simulink model "rockets_v2"  (R2020a)
settings: Solver=VariableStepAuto  StartTime=0.0  StopTime=10  RelTol=1e-3
undefined symbols (not defined in the file): Earth, F_z, length_rocket, mass_rocket, WGS84
libraries: shared6dof x1, aerolibtransform2 x1, aerolibfltsims x1, vrlib x1, sharedtransform x1
settings Model: PacingRate=0.890000  Creator=Benjamin_de_worsop  LastModifiedBy=Benjamin_de_worsop

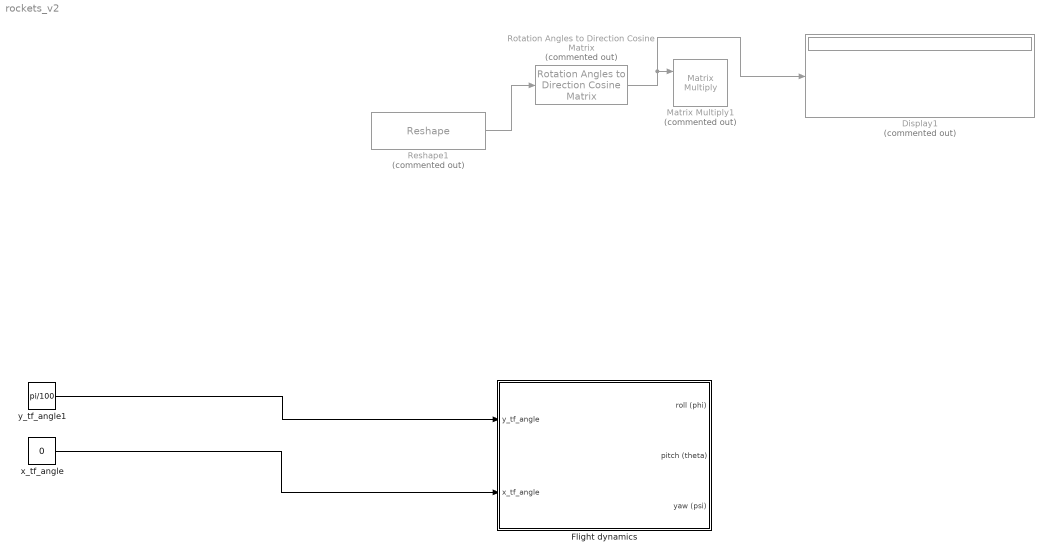
== system rockets_v2 ==
  Display1 : Display  Commented=on
  Flight dynamics : Subsystem
  Matrix Multiply1 : Product  Commented=on  Multiplication=Matrix(*)
  Reshape1 : Reshape  Commented=on  OutputDimensionality=Customize  OutputDimensions=[1, 3]
  Rotation Angles to Direction Cosine Matrix : sharedtransform/Rotation Angles to Direction Cosine Matrix  Commented=on  rotationOrder=YXZ  aMode=aMode
      settings: SourceProductBaseCode=AE,PW,MT,VE,VP
  x_tf_angle : Constant  Value=0
  y_tf_angle1 : Constant  Value=pi/100
  wires:
  Rotation Angles to Direction Cosine Matrix/1 -> Display1/1, Matrix Multiply1/1
  Reshape1/1 -> Rotation Angles to Direction Cosine Matrix/1
  y_tf_angle1/1 -> Flight dynamics/1(y_tf_angle)
  x_tf_angle/1 -> Flight dynamics/2(x_tf_angle)

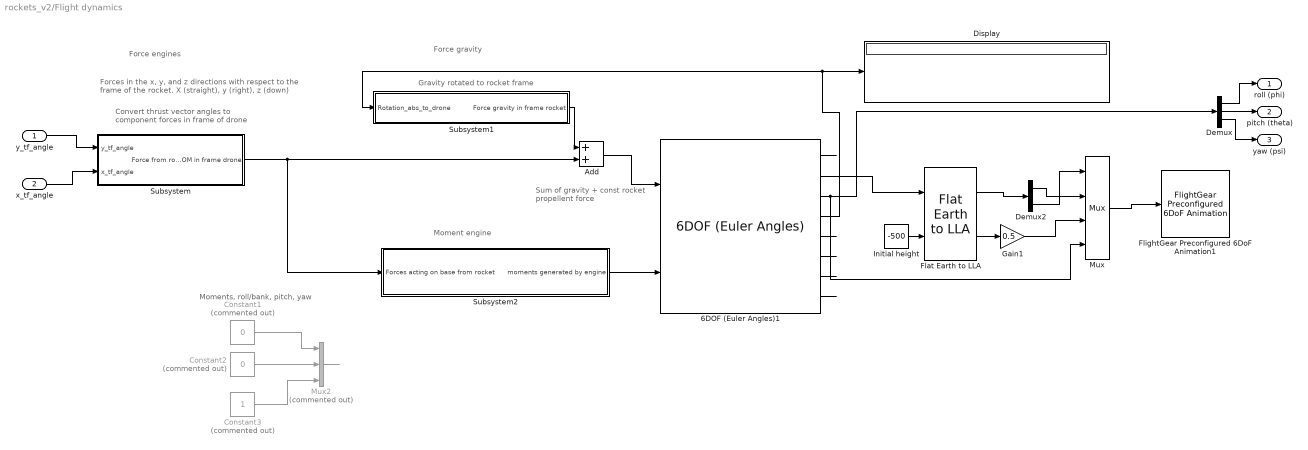
== system rockets_v2/Flight dynamics ==
  note: Convert thrust vector angles to component forces in frame of drone
  note: Moment engine
  note: Sum of gravity + const rocket propellent force
  note: Gravity rotated to rocket frame
  note: Forces in the x, y, and z directions with respect to the frame of the rocket. X (straight), y (right), z (down)
  note: Moments, roll/bank, pitch, yaw
  note: Force engines
  note: Force gravity
  y_tf_angle : Inport
  x_tf_angle : Inport  Port=2
  6DOF (Euler Angles)1 : shared6dof/6DOF (Euler Angles)  units=Metric (MKS)  mtype=Fixed  rep=Euler Angles  xme_0=[-122.482, 37.6655, 400]  Vm_0=[0 0 0]  eul_0=[0 0 0]  pm_0=[0 0 0]  mass_0=1  mass_e=0.5  mass_f=2.0  inertia=eye(3)  inertia_e=eye(3)  inertia_f=2*eye(3)  k_quat=1.0  vre_flag=on  abi_flag=off  aMode=0  xme_statename=''  Vm_statename=''  eul_statename=''  quat_statename=''  pm_statename=''  mass_statename=''
      settings: SourceProductBaseCode=AE,PW,MT,VE,VP
  Add : Sum
  Constant1 : Constant  Commented=on  Value=0
  Constant2 : Constant  Commented=on  Value=0
  Constant3 : Constant  Commented=on
  Demux : Demux  Outputs=3
  Demux2 : Demux  Outputs=2
  Display : Display
  Flat Earth to LLA : aerolibtransform2/Flat Earth to LLA  units=Metric (MKS)  ptype=Earth (WGS84)  F=1/298.257223563  R=6378137  refPosPort=off  LL0=[0 10]  psi=0
  FlightGear Preconfigured 6DoF Animation1 : aerolibfltsims/FlightGear Preconfigured 6DoF Animation  xFlightGearVersion=v2019.1  DestinationIpAddress=127.0.0.1  DestinationPort=5502  SampleTime=1/30  packetVersion=24
  Gain1 : Gain  Gain=0.5
  Initial height : Constant  Value=-500
  Mux : Mux
  Mux2 : Mux  Commented=on  Inputs=3
  Subsystem : Subsystem
  Subsystem1 : Subsystem
  Subsystem2 : Subsystem
  roll (phi) : Outport
  pitch (theta) : Outport  Port=2
  yaw (psi) : Outport  Port=3
  wires:
  Demux2/1 -> Mux/2
  Flat Earth to LLA/1 -> Demux2/1
  Gain1/1 -> Mux/3
  Demux2/2 -> Mux/1
  Subsystem/1(Force from rocket COM in frame drone) -> Add/2, Subsystem2/1(Forces acting on base from rocket)
  Initial height/1 -> Flat Earth to LLA/2
  6DOF (Euler Angles)1/8 -> ?
  6DOF (Euler Angles)1/6 -> ?
  Mux/1 -> FlightGear Preconfigured 6DoF Animation1/1
  Flat Earth to LLA/2 -> Gain1/1
  6DOF (Euler Angles)1/2 -> Flat Earth to LLA/1
  6DOF (Euler Angles)1/5 -> ?
  6DOF (Euler Angles)1/4 -> Display/1, Subsystem1/1(Rotation_abs_to_drone)
  6DOF (Euler Angles)1/3 -> Demux/1, Mux/4
  Subsystem2/1(moments generated by engine) -> 6DOF (Euler Angles)1/2
  x_tf_angle/1 -> Subsystem/2(x_tf_angle)
  Constant1/1 -> Mux2/1
  Constant3/1 -> Mux2/3
  Constant2/1 -> Mux2/2
  Subsystem1/1(Force gravity in frame rocket) -> Add/1
  Add/1 -> 6DOF (Euler Angles)1/1
  6DOF (Euler Angles)1/7 -> ?
  Mux2/1 -> ?
  6DOF (Euler Angles)1/1 -> ?
  y_tf_angle/1 -> Subsystem/1(y_tf_angle)
  Demux/1 -> roll (phi)/1
  Demux/2 -> pitch (theta)/1
  Demux/3 -> yaw (psi)/1

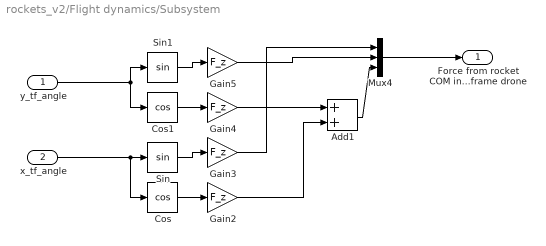
== system rockets_v2/Flight dynamics/Subsystem ==
  y_tf_angle : Inport
  x_tf_angle : Inport  Port=2
  Add1 : Sum
  Cos : Trigonometry  Operator=cos
  Cos1 : Trigonometry  Operator=cos
  Gain{2..5} (4 alike) : Gain  Gain=F_z
  Mux4 : Mux  Inputs=3
  Sin : Trigonometry
  Sin1 : Trigonometry
  Force from rocket COM in frame drone : Outport
  wires:
  Gain4/1 -> Add1/1
  y_tf_angle/1 -> Sin1/1, Cos1/1
  x_tf_angle/1 -> Cos/1, Sin/1
  Cos1/1 -> Gain4/1
  Add1/1 -> Mux4/3
  Sin1/1 -> Gain5/1
  Cos/1 -> Gain2/1
  Gain3/1 -> Mux4/1
  Gain2/1 -> Add1/2
  Gain5/1 -> Mux4/2
  Sin/1 -> Gain3/1
  Mux4/1 -> Force from rocket COM in frame drone/1

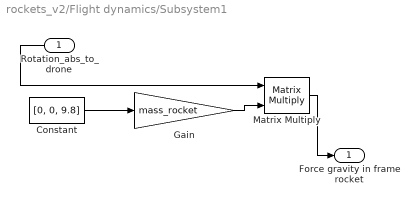
== system rockets_v2/Flight dynamics/Subsystem1 ==
  Rotation_abs_to_drone : Inport
  Constant : Constant  Value=[0, 0, 9.8]
  Gain : Gain  Gain=mass_rocket
  Matrix Multiply : Product  Multiplication=Matrix(*)
  Force gravity in frame rocket : Outport
  wires:
  Matrix Multiply/1 -> Force gravity in frame rocket/1
  Gain/1 -> Matrix Multiply/2
  Constant/1 -> Gain/1
  Rotation_abs_to_drone/1 -> Matrix Multiply/1

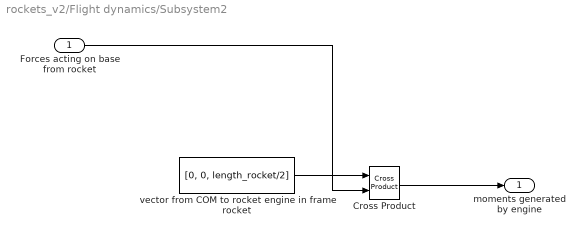
== system rockets_v2/Flight dynamics/Subsystem2 ==
  Forces acting on base from rocket : Inport
  Cross Product : vrlib/Utilities/Cross Product
  vector from COM to rocket engine in frame rocket : Constant  Value=[0, 0, length_rocket/2]
  moments generated by engine : Outport
  wires:
  vector from COM to rocket engine in frame rocket/1 -> Cross Product/1
  Forces acting on base from rocket/1 -> Cross Product/2
  Cross Product/1 -> moments generated by engine/1
